simulink model "model_main3"  (R2024b)
settings: Solver=ode4  StartTime=0.0  StopTime=1000  FixedStep=dt  RelTol=1e-3
values from neighbouring files (symbols this model uses):
  dt = 0.01    [model_init.m]
  Iws = diag([1 1 1 1])*0.2274    [model_init.m]
  m_tot = 3300    [model_init.m]
  Omega1_init = 1500*rpm2rad    (= 157.079632679)    [model_init.m]
  Omega2_init = 2500*rpm2rad    (= 261.799387799)    [model_init.m]
  Omega3_init = 1500*rpm2rad    (= 157.079632679)    [model_init.m]
  Omega4_init = 2500*rpm2rad    (= 261.799387799)    [model_init.m]
  qb0 = angle2quat(ag0(1),ag0(2),ag0(3),'ZYX')'    [model_init.m]
  rad2rpm = 1/rpm2rad    (= 9.54929658551)    [model_init.m]
  RCS_F = 1.0    (= 1)    [model_init.m]
  RCS_Pos = [RCS1_POS , RCS2_POS , RCS3_POS , RCS4_POS ,            RCS5_POS , RCS6_POS , RCS7_POS , RCS8_POS ,            RCS9_POS , RCS10_POS, RCS11_POS, RCS12_POS,            RCS13_POS, RCS14_POS, RCS15_POS, RCS16_POS]    [model_init.m]
  RCS_PWM_Freq = 0.1    [model_init.m]
  RCS_Sampling_time = 0.01    [model_init.m]
  RCS_THR_vec = [RCS1_THR , RCS2_THR , RCS3_THR , RCS4_THR,                 RCS5_THR , RCS6_THR , RCS7_THR , RCS8_THR,                 RCS9_THR , RCS10_THR, RCS11_THR, RCS12_THR,                 RCS13_THR, RCS14_THR, RCS15_THR, RCS16_THR]    [model_init.m]
  RW_As = [RW1_Axis,RW2_Axis,RW3_Axis,RW4_Axis]    [model_init.m]
  RW_Omegad_max = RW_t_max    (= 0.5)    [model_init.m]
  SC_Ib = [1843.56  -0.0019  -803.89 ... (first row only)    [model_init.m]
  SC_Kepler = [(6371.2+600)*1000, 0.00221, 0*pi/180, 0*pi/180, 0, deg2rad(270)]    [model_init.m]
  wb0 = deg2rad([-0.3 -0.1 0.2])'    [model_init.m]
undefined symbols (not defined in the file or in its folder): RS_Max_Speed, TC_Kepler
libraries: simulink x16, simulink_extras x9, sharedtransform x6, aerolibutil x4
settings Model: PacingRate=1.100000  Creator=yhj2019  LastModifiedBy=ASCL
settings DebuggingCC: UnderSpecifiedDimensionMsg=warning
settings RTWCC: GPUComputeCapability=3.5

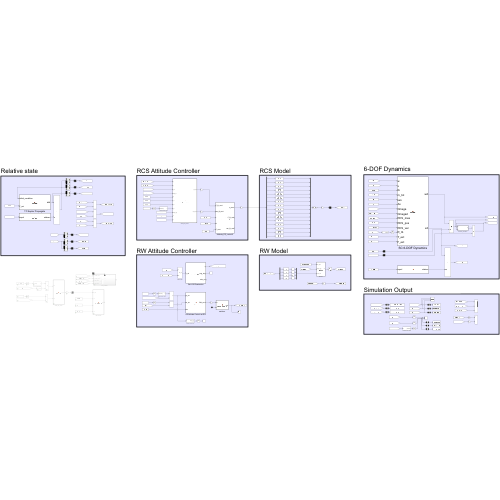
[thumbnail: Simulink's stored preview of the top-level diagram]
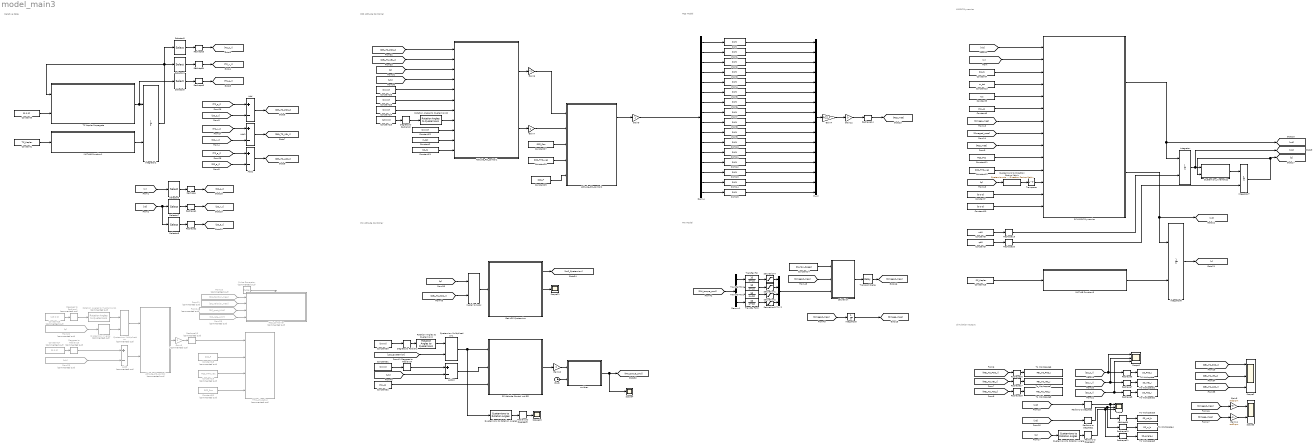
== system model_main3 ==
  note: Relative state
  note: RW Model
  note: RW Attitude Controller
  note: RCS Model
  note: Simulation Output
  note: RCS Attitude Controller
  note: 6-DOF Dynamics
  Add{,1..2,10} (4 alike) : Sum  Inputs=+-
  Add3 : Sum  Commented=on  Inputs=+-
  Attitude_PD_control : MATLAB Function  Commented=on  TreatAsAtomicUnit=on
  Attitude_PD_control1 : MATLAB Function  TreatAsAtomicUnit=on
  Attitude_PD_control2 : MATLAB Function  TreatAsAtomicUnit=on
  Clock : Clock
  Constant1 : Constant  Value=TC_Kepler
  Constant{3,7,10,22,24..25} (6 alike) : Constant  Value=[0 0 0]'
  Constant11 : Constant  Value=RCS_Pos
  Constant12 : Constant  Value=RCS_THR_vec
  Constant13 : Constant  Value=m_tot
  Constant14 : Constant  Value=RS_Max_Speed
  Constant15 : Constant  Value=SC_Kepler
  Constant16 : Constant  Commented=on  Value=[45 0 0]
  Constant17 : Constant  Commented=on  Value=[0 0 0]
  Constant18 : Constant  Commented=on  Value=RCS_F
  Constant19 : Constant  Commented=on  Value=RCS_THR_vec
  Constant2 : Constant  Value=m_tot
  Constant20 : Constant  Commented=on  Value=RCS_Pos
  Constant21 : Constant  Value=SC_Ib
  Constant23 : Constant  Value=[45 0 0]
  Constant26 : Constant  Value=[3 0 0]'
  Constant27 : Constant  Value=RCS_Pos
  Constant28 : Constant  Value=RCS_THR_vec
  Constant29 : Constant  Value=RCS_F
  Constant30 : Constant  Value=[0 0 0]
  Constant31 : Constant  Value=[0 0 0]
  Constant32 : Constant  Value=RW_As
  Constant4 : Constant  Value=SC_Ib
  Constant5 : Constant  Value=Iws
  Constant6 : Constant  Value=RW_As
  Constant8 : Constant  Value=wb0
  Constant9 : Constant  Value=qb0
  Degrees to Radians : simulink_extras/Transformations/Degrees to Radians
  Degrees to Radians1 : simulink_extras/Transformations/Degrees to Radians  Commented=on
  Degrees to Radians2 : simulink_extras/Transformations/Degrees to Radians
  Degrees to Radians3 : simulink_extras/Transformations/Degrees to Radians  Commented=on
  Degrees to Radians4 : simulink_extras/Transformations/Degrees to Radians
  Demux : Demux  Outputs=16
  Demux1 : Demux
  From10 : From  Commented=on  GotoTag=SC_Position_mea  TagVisibility=global
  From11 : From  Commented=on  GotoTag=SC_Velocity_mea  TagVisibility=global
  From22 : From  Commented=on  GotoTag=q
  From23 : From  Commented=on  GotoTag=wb
  From24 : From  Commented=on  GotoTag=SC_quat_LVLH  TagVisibility=global
  From25 : From  Commented=on  GotoTag=SC_rate_LVLH  TagVisibility=global
  Gain10 : Gain
  Gain11 : Gain  Gain=rad2rpm
  Gain12 : Gain  Gain=0
  Gain4 : Gain  Gain=RCS_F
  Gain5 : Gain  Commented=on
  Gain6 : Gain  Gain=-1
  Gain7 : Gain
  Gain8 : Gain  Gain=rad2rpm
  Gain9 : Gain
  Get LOS Quaternion : MATLAB Function  TreatAsAtomicUnit=on
  Inetial to body : aerolibutil/Quaternion Rotation
  Integrator : Integrator  InitialConditionSource=external  InitialCondition=wb0
  Integrator1 : Integrator  InitialConditionSource=external  InitialCondition=[-7000 0 0 0 -9.175045 0 5233.5]'
  Integrator3 : Integrator  InitialCondition=[Omega1_init Omega2_init Omega3_init Omega4_init]'
  Integrator7 : Integrator  InitialConditionSource=external
  Integrator8 : Integrator  InitialConditionSource=external  InitialCondition=[-7000 0 0 0 -9.175045 0 5233.5]'
  MATLAB Function1 : MATLAB Function  TreatAsAtomicUnit=on
  MATLAB Function3 : MATLAB Function  TreatAsAtomicUnit=on
  Mux1 : Mux
  Mux2 : Mux  Inputs=16
  PWM{,1..15} (16 alike) : simulink/Discontinuities/PWM  DisableCoverage=on  Period=RCS_PWM_Freq  InitialDelay=0  DisallowZeroDutyCycle=off  RunAtFixedTimeIntervals=on  SampleTime=RCS_Sampling_time
  Pulse Generator : DiscretePulseGenerator  Commented=on  PulseType=Time based  Period=0.2  PulseWidth=50
  Quaternion Inverse : aerolibutil/Quaternion Inverse  Commented=on
  Quaternion Multiplication : aerolibutil/Quaternion Multiplication  Commented=on
  Quaternion Multiplication1 : aerolibutil/Quaternion Multiplication
  Quaternion_Kinematics : MATLAB Function  TreatAsAtomicUnit=on
  Quaternions to Direction Cosine Matrix : sharedtransform/Quaternions to  Direction Cosine Matrix  aMode=aMode
      settings: LibrarySourceBlock=|
      | aerolibtransform2/Quaternions to
      | Direction Cosine Matrix
  Quaternions to Rotation Angles : sharedtransform/Quaternions to Rotation Angles  rotationOrder=ZYX  aMode=aMode
  Quaternions to Rotation Angles1 : sharedtransform/Quaternions to Rotation Angles  rotationOrder=ZYX  aMode=aMode
  RCS_Controller : Subsystem  Commented=on
  Radians to Degrees{,1..2,5} (4 alike) : simulink_extras/Transformations/Radians to Degrees
  Reshape{,1..5,14,19..20} (9 alike) : Reshape  OutputDimensionality=Column vector (2-D)
  Reshape{6..11,16..18} (9 alike) : Reshape  OutputDimensionality=Row vector (2-D)
  Reshape15 : Reshape  Commented=on  OutputDimensionality=Column vector (2-D)
  Rotation Angles to Quaternions : sharedtransform/Rotation Angles to Quaternions  rotationOrder=ZYX  aMode=aMode
  Rotation Angles to Quaternions1 : sharedtransform/Rotation Angles to Quaternions  Commented=on  rotationOrder=ZYX  aMode=aMode
  Rotation Angles to Quaternions2 : sharedtransform/Rotation Angles to Quaternions  rotationOrder=ZYX  aMode=aMode
  SC 6-DOF Dynamics : MATLAB Function  TreatAsAtomicUnit=on
  SS Attitude Control wrt ECI : MATLAB Function  TreatAsAtomicUnit=on
  Saturation{1..4} (4 alike) : Saturate  UpperLimit=RW_Omegad_max  LowerLimit=-RW_Omegad_max
  Scope : Scope  NumInputPorts=3
  Scope1 : Scope  NumInputPorts=3
  Scope11 : Scope
  Scope13 : Scope
  Scope2 : Scope  NumInputPorts=3
  Scope3 : Scope  NumInputPorts=2
  Scope4 : Scope
  Selector3 : Selector  InputPortWidth=6  IndexOptions=Index vector (dialog)  Indices=[1 2 3]  OutputSizes=1
  Selector4 : Selector  InputPortWidth=6  IndexOptions=Index vector (dialog)  Indices=[4 5 6]  OutputSizes=1
  Selector5 : Selector  InputPortWidth=6  IndexOptions=Index vector (dialog)  Indices=[4 5 6]  OutputSizes=1
  Selector6 : Selector  InputPortWidth=6  IndexOptions=Index vector (dialog)  Indices=[1 2 3]  OutputSizes=1
  Selector7 : Selector  InputPortWidth=6  IndexOptions=Index vector (dialog)  Indices=[1 2 3]  OutputSizes=1
  Selector8 : Selector  InputPortWidth=6  IndexOptions=Index vector (dialog)  Indices=[4 5 6]  OutputSizes=1
  TC Kepler Propagate : MATLAB Function  TreatAsAtomicUnit=on
  THR_Allocation : MATLAB Function  Commented=on  TreatAsAtomicUnit=on
  To Workspace : ToWorkspace  VariableName=SS_POS_I  SampleTime=-1
      settings: Save2DSignal=2-D array (concatenate along first dimension)
  To Workspace1 : ToWorkspace  VariableName=SS_VEL_I  SampleTime=-1
      settings: Save2DSignal=2-D array (concatenate along first dimension)
  To Workspace2 : ToWorkspace  VariableName=SS_ACC_I  SampleTime=-1
      settings: Save2DSignal=2-D array (concatenate along first dimension)
  To Workspace3 : ToWorkspace  VariableName=SS_wd_b  SampleTime=-1
      settings: Save2DSignal=2-D array (concatenate along first dimension)
  To Workspace4 : ToWorkspace  VariableName=SS_w_b  SampleTime=-1
      settings: Save2DSignal=2-D array (concatenate along first dimension)
  To Workspace5 : ToWorkspace  VariableName=SS_angle_I  SampleTime=-1
      settings: Save2DSignal=2-D array (concatenate along first dimension)
  To Workspace6 : ToWorkspace  VariableName=REL_TS_POS_I  SampleTime=-1
      settings: Save2DSignal=2-D array (concatenate along first dimension)
  To Workspace7 : ToWorkspace  VariableName=REL_TS_VEL_I  SampleTime=-1
      settings: Save2DSignal=2-D array (concatenate along first dimension)
  To Workspace8 : ToWorkspace  VariableName=REL_TS_ACC_I  SampleTime=-1
      settings: Save2DSignal=2-D array (concatenate along first dimension)
  Transfer Fcn{,1..3} (4 alike) : TransferFcn  Numerator=[10]  Denominator=[1 10]
  Transport Delay : TransportDelay  DelayTime=dt  InitialOutput=[0 0 0 0]'
  Transpose : Math  Operator=transpose
  saturation : MATLAB Function  TreatAsAtomicUnit=on
  swicher : MATLAB Function  TreatAsAtomicUnit=on
  wires:
  Constant1/1 -> MATLAB Function1/1(kepel)
  TC Kepler Propagate/1(dfdt) -> Selector5/1, Integrator1/1
  MATLAB Function1/1(statvec) -> Integrator1/2
  Integrator1/1 -> Selector3/1, TC Kepler Propagate/1(initial_condition), Selector4/1
  Constant3/1 -> TC Kepler Propagate/2(F_eci)
  Selector5/1 -> Reshape5/1
  Selector4/1 -> Reshape4/1
  Selector3/1 -> Reshape3/1
  Reshape4/1 -> [TS_v_I]
  Reshape5/1 -> [TS_a_I]
  Reshape3/1 -> [TS_p_I]
  Reshape6/1 -> To Workspace/1
  Reshape7/1 -> To Workspace1/1
  Reshape8/1 -> To Workspace2/1
  [TS_p_I] -> Add/1
  [SS_p_I] -> Add/2
  [SS_v_I] -> Add1/2
  [TS_v_I] -> Add1/1
  [SS_a_I] -> Add2/2
  [TS_a_I] -> Add2/1
  Add/1 -> [REL_TS_POS_I]
  Add1/1 -> [REL_TS_VEL_I]
  Add2/1 -> [REL_TS_ACC_I]
  Constant4/1 -> SC 6-DOF Dynamics/3(Ib)
  Constant5/1 -> SC 6-DOF Dynamics/5(Iws)
  SC 6-DOF Dynamics/1(wd) -> Integrator/1, [wd]
  [wb] -> SC 6-DOF Dynamics/1(w)
  Constant6/1 -> SC 6-DOF Dynamics/6(As)
  Constant7/1 -> SC 6-DOF Dynamics/13(T_ext)
  [Omega_mea] -> SC 6-DOF Dynamics/7(Omega)
  [Omegad_mea] -> SC 6-DOF Dynamics/8(Omegad)
  Quaternion_Kinematics/1(qd) -> Integrator7/1
  Constant8/1 -> Reshape19/1
  Constant9/1 -> Reshape20/1
  Quaternions to Rotation Angles/1 -> Radians to Degrees2/1
  [wd] -> Radians to Degrees/1
  [wb] -> Radians to Degrees1/1
  Radians to Degrees/1 -> Reshape9/1, Scope/1
  Radians to Degrees1/1 -> Reshape10/1, Scope/2
  Radians to Degrees2/1 -> Reshape11/1, Scope/3
  [q] -> Quaternions to Rotation Angles/1
  Constant10/1 -> SC 6-DOF Dynamics/14(F_ext)
  Constant13/1 -> SC 6-DOF Dynamics/4(m_tot)
  [q] -> Quaternions to Direction Cosine Matrix/1
  Quaternions to Direction Cosine Matrix/1 -> Transpose/1
  [SS_v_I] -> Scope1/2, Reshape7/1
  Transpose/1 -> SC 6-DOF Dynamics/12(R_Ib)
  Reshape9/1 -> To Workspace3/1
  Reshape10/1 -> To Workspace4/1
  Reshape11/1 -> To Workspace5/1
  Constant15/1 -> MATLAB Function3/1(kepel)
  MATLAB Function3/1(statvec) -> Integrator8/2
  SC 6-DOF Dynamics/2(xd) -> Integrator8/1, [xd]
  Integrator8/1 -> [x]
  Selector8/1 -> Reshape2/1
  Selector6/1 -> Reshape/1
  [xd] -> Selector8/1, Selector7/1
  [x] -> Selector6/1
  Selector7/1 -> Reshape1/1
  [x] -> SC 6-DOF Dynamics/2(x)
  Constant11/1 -> SC 6-DOF Dynamics/10(RCS_pos)
  Constant12/1 -> SC 6-DOF Dynamics/11(RCS_vec)
  Demux/1 -> PWM/1
  Demux/2 -> PWM1/1
  Demux/3 -> PWM2/1
  Demux/4 -> PWM3/1
  Demux/8 -> PWM7/1
  Demux/5 -> PWM4/1
  Demux/6 -> PWM5/1
  Demux/7 -> PWM6/1
  Demux/14 -> PWM13/1
  Demux/13 -> PWM12/1
  Demux/15 -> PWM14/1
  Demux/12 -> PWM11/1
  Demux/16 -> PWM15/1
  Demux/9 -> PWM8/1
  Demux/10 -> PWM9/1
  Demux/11 -> PWM10/1
  Reshape14/1 -> [RCS_mea]
  PWM/1 -> Mux2/1
  Mux2/1 -> Gain4/1
  PWM1/1 -> Mux2/2
  PWM2/1 -> Mux2/3
  PWM3/1 -> Mux2/4
  PWM4/1 -> Mux2/5
  PWM5/1 -> Mux2/6
  PWM6/1 -> Mux2/7
  PWM7/1 -> Mux2/8
  PWM8/1 -> Mux2/9
  PWM9/1 -> Mux2/10
  PWM10/1 -> Mux2/11
  PWM11/1 -> Mux2/12
  PWM12/1 -> Mux2/13
  PWM13/1 -> Mux2/14
  PWM14/1 -> Mux2/15
  PWM15/1 -> Mux2/16
  [RCS_mea] -> SC 6-DOF Dynamics/9(RCS_mea)
  Gain4/1 -> Gain12/1
  From11/1 -> RCS_Controller/2(SC_Velocity_mea)
  From25/1 -> RCS_Controller/4(SC_rate_LVLH)
  From10/1 -> RCS_Controller/1(SC_Position_mea)
  Pulse Generator/1 -> RCS_Controller/Trigger
  From24/1 -> RCS_Controller/3(SC_quat_LVLH)
  From22/1 -> Quaternion Inverse/1
  Degrees to Radians3/1 -> Add3/1
  Constant18/1 -> THR_Allocation/2(F_on)
  Quaternion Inverse/1 -> Quaternion Multiplication/2
  Quaternion Multiplication/1 -> Attitude_PD_control/1(q_err)
  Constant20/1 -> THR_Allocation/4(r_thr)
  Reshape15/1 -> THR_Allocation/1(tau_cmd)
  From23/1 -> Add3/2
  Attitude_PD_control/1(u_torq) -> Gain5/1
  Degrees to Radians1/1 -> Rotation Angles to Quaternions1/1
  Constant17/1 -> Degrees to Radians3/1
  Rotation Angles to Quaternions1/1 -> Quaternion Multiplication/1
  Constant19/1 -> THR_Allocation/3(f)
  Gain5/1 -> Reshape15/1
  Add3/1 -> Attitude_PD_control/2(w_err)
  Constant16/1 -> Degrees to Radians1/1
  Reshape/1 -> [SS_p_I]
  Reshape1/1 -> [SS_v_I]
  Reshape2/1 -> [SS_a_I]
  [REL_TS_POS_I] -> Reshape16/1
  [REL_TS_VEL_I] -> Reshape17/1
  [REL_TS_ACC_I] -> Reshape18/1
  Reshape16/1 -> To Workspace6/1
  Reshape17/1 -> To Workspace7/1
  Reshape18/1 -> To Workspace8/1
  Attitude_PD_control1/1(F_B_cmd) -> Gain6/1
  Attitude_PD_control1/2(tau_B_cmd) -> Gain7/1
  Attitude_PD_control2/1(u_pwm) -> Gain9/1
  Constant21/1 -> Attitude_PD_control1/11(J)
  Constant2/1 -> Attitude_PD_control1/10(m)
  Constant22/1 -> Attitude_PD_control1/9(omega_d_B)
  Constant23/1 -> Degrees to Radians2/1
  Degrees to Radians2/1 -> Rotation Angles to Quaternions2/1
  Rotation Angles to Quaternions2/1 -> Attitude_PD_control1/8(q_d)
  Constant24/1 -> Attitude_PD_control1/7(a_d)
  Constant25/1 -> Attitude_PD_control1/6(v_d)
  Constant26/1 -> Attitude_PD_control1/5(r_d)
  [wb] -> Attitude_PD_control1/4(omega_B)
  [q] -> Attitude_PD_control1/3(q_IB)
  [REL_TS_POS_I] -> Attitude_PD_control1/1(r_I)
  Gain6/1 -> Attitude_PD_control2/1(F_B_cmd)
  Constant27/1 -> Attitude_PD_control2/3(r)
  Constant28/1 -> Attitude_PD_control2/4(d)
  Constant29/1 -> Attitude_PD_control2/5(F_max)
  [REL_TS_POS_I] -> Scope2/1
  [REL_TS_VEL_I] -> Scope2/2
  [REL_TS_ACC_I] -> Scope2/3
  Gain7/1 -> Attitude_PD_control2/2(tau_B_cmd)
  [REL_TS_VEL_I] -> Attitude_PD_control1/2(v_I)
  [wb] -> Add10/2
  Clock/1 -> swicher/2(t)
  Rotation Angles to Quaternions/1 -> Quaternion Multiplication1/1
  Quaternions to Rotation Angles1/1 -> Radians to Degrees5/1
  Get LOS Quaternion/2(ang_deg) -> Scope11/1
  Radians to Degrees5/1 -> Scope13/1
  Degrees to Radians4/1 -> Add10/1
  Constant32/1 -> SS Attitude Control wrt ECI/3(As)
  Degrees to Radians/1 -> Rotation Angles to Quaternions/1
  Quaternion Multiplication1/1 -> SS Attitude Control wrt ECI/1(q_err), Quaternions to Rotation Angles1/1
  Get LOS Quaternion/1(q) -> [LoS_Quaternion]
  Add10/1 -> SS Attitude Control wrt ECI/2(w_err)
  [LoS_Quaternion] -> Quaternion Multiplication1/2
  Constant30/1 -> Degrees to Radians/1
  Constant31/1 -> Degrees to Radians4/1
  [q] -> Inetial to body/1
  Inetial to body/1 -> Get LOS Quaternion/1(r_rel)
  SS Attitude Control wrt ECI/1(RW_cmd) -> Gain10/1
  [REL_TS_POS_I] -> Inetial to body/2
  Gain9/1 -> Demux/1
  Gain10/1 -> swicher/1(in)
  Gain8/1 -> Scope3/1
  Gain11/1 -> Scope3/2
  Reshape19/1 -> Integrator/2
  Reshape20/1 -> Integrator7/2
  Gain12/1 -> Reshape14/1
  Demux1/1 -> Transfer Fcn/1
  Demux1/4 -> Transfer Fcn3/1
  Demux1/2 -> Transfer Fcn1/1
  Demux1/3 -> Transfer Fcn2/1
  Transfer Fcn/1 -> Saturation4/1
  Transfer Fcn1/1 -> Saturation1/1
  Transfer Fcn2/1 -> Saturation2/1
  Transfer Fcn3/1 -> Saturation3/1
  saturation/1(res) -> Transport Delay/1
  [Omegad_mea] -> Integrator3/1
  Integrator3/1 -> [Omega_mea]
  Integrator/1 -> [wb], Quaternion_Kinematics/1(w)
  Integrator7/1 -> [q], Quaternion_Kinematics/2(q)
  swicher/1(out) -> Scope4/1, [RW_torque_cmd]
  [Omegad_mea] -> Gain8/1
  [Omega_mea] -> Gain11/1
  [RW_torque_cmd] -> Demux1/1
  Transport Delay/1 -> [Omegad_mea]
  Saturation3/1 -> Mux1/4
  Saturation1/1 -> Mux1/2
  Saturation4/1 -> Mux1/1
  Saturation2/1 -> Mux1/3
  Mux1/1 -> saturation/3(torque_cmd)
  [Omegad_mea] -> saturation/2(Omega_mea)
  Constant14/1 -> saturation/1(max_speed)
  [SS_p_I] -> Scope1/1, Reshape6/1
  [SS_a_I] -> Scope1/3, Reshape8/1

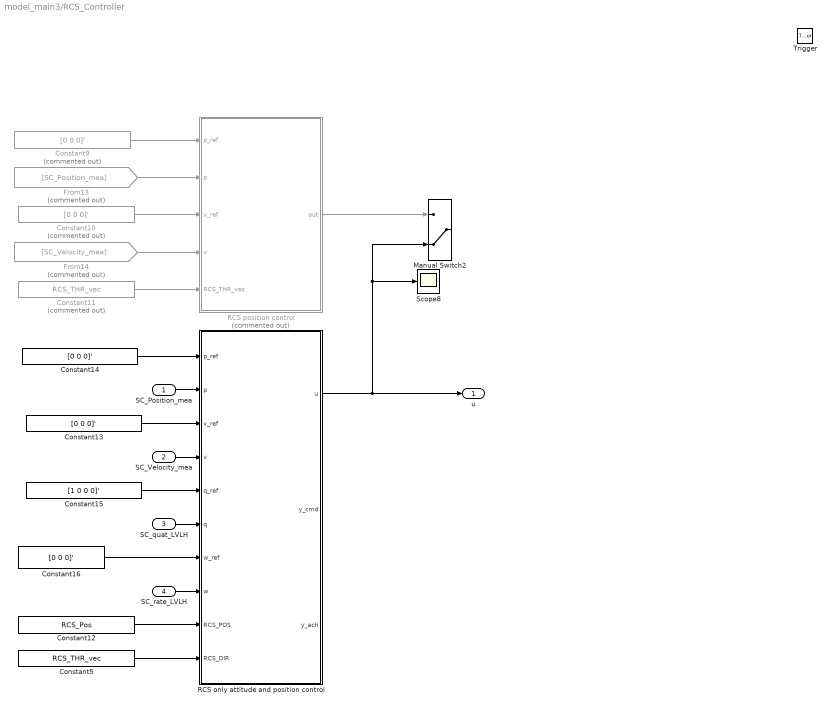
== system model_main3/RCS_Controller ==
  SC_Position_mea : Inport
  SC_Velocity_mea : Inport  Port=2
  SC_quat_LVLH : Inport  Port=3
  SC_rate_LVLH : Inport  Port=4
  Trigger : TriggerPort  TriggerType=either  VariantControl=(inherit)  PortDimensions=1
  Constant10 : Constant  Commented=on  Value=[0 0 0]'
  Constant11 : Constant  Commented=on  Value=RCS_THR_vec
  Constant12 : Constant  Value=RCS_Pos
  Constant13 : Constant  Value=[0 0 0]'
  Constant14 : Constant  Value=[0 0 0]'
  Constant15 : Constant  Value=[1 0 0 0]'
  Constant16 : Constant  Value=[0 0 0]'
  Constant5 : Constant  Value=RCS_THR_vec
  Constant9 : Constant  Commented=on  Value=[0 0 0]'
  From13 : From  Commented=on  GotoTag=SC_Position_mea  TagVisibility=global
  From14 : From  Commented=on  GotoTag=SC_Velocity_mea  TagVisibility=global
  Manual Switch2 : ManualSwitch  CurrentSetting=0
  RCS only attitude and position control : MATLAB Function  TreatAsAtomicUnit=on
  RCS position control : MATLAB Function  Commented=on  TreatAsAtomicUnit=on
  Scope8 : Scope
  u : Outport
  wires:
  Constant5/1 -> RCS only attitude and position control/10(RCS_DIR)
  SC_quat_LVLH/1 -> RCS only attitude and position control/6(q)
  Constant12/1 -> RCS only attitude and position control/9(RCS_POS)
  SC_rate_LVLH/1 -> RCS only attitude and position control/8(w)
  SC_Velocity_mea/1 -> RCS only attitude and position control/4(v)
  From13/1 -> RCS position control/2(p)
  RCS only attitude and position control/1(u) -> Manual Switch2/2, Scope8/1, u/1
  Constant13/1 -> RCS only attitude and position control/3(v_ref)
  Constant15/1 -> RCS only attitude and position control/5(q_ref)
  RCS position control/1(out) -> Manual Switch2/1
  Constant16/1 -> RCS only attitude and position control/7(w_ref)
  Constant10/1 -> RCS position control/3(v_ref)
  Constant9/1 -> RCS position control/1(p_ref)
  Constant11/1 -> RCS position control/5(RCS_THR_vec)
  SC_Position_mea/1 -> RCS only attitude and position control/2(p)
  Constant14/1 -> RCS only attitude and position control/1(p_ref)
  From14/1 -> RCS position control/4(v)

== matlab function model_main3/Attitude_PD_control1 ==
  settings: updateMethod=DISCRETE
  data: F_B_cmd output; r_I input; v_I input; q_IB input; omega_B input; r_d input; v_d input; a_d input; q_d input; omega_d_B input; m input; J input; tau_B_cmd output
function [F_B_cmd, tau_B_cmd] = CTRL_WRENCH_6DOF( ...
    r_I, v_I, q_IB, omega_B, ...
    r_d, v_d, a_d, q_d, omega_d_B, ...
    m, J)
%#codegen
% ============================================================
% Controller block
% Input :
%   r_I      [3x1] current position in inertial frame
%   v_I      [3x1] current velocity in inertial frame
%   q_IB     [4x1] quaternion [qw qx qy qz], Body -> Inertial
%   omega_B  [3x1] current angular velocity in body frame
%
%   r_d      [3x1] desired position in inertial frame
%   v_d      [3x1] desired velocity in inertial frame
%   a_d      [3x1] desired acceleration in inertial frame
%   q_d      [4x1] desired quaternion, Body -> Inertial
%   omega_d_B[3x1] desired angular velocity in body frame
%
%   m        scalar mass
%   J        [3x3] inertia matrix in body frame
%
% Output:
%   F_B_cmd    [3x1] desired total body force
%   tau_B_cmd  [3x1] desired total body torque
% ============================================================

    % -------------------------
    % Quaternion normalize
    % -------------------------
    q_IB = quat_normalize(q_IB);
    q_d  = quat_normalize(q_d);

    % -------------------------
    % Gains (example)
    % -------------------------
    Kp_r = diag([0.010, 0.010, 0.010]);   % position gain
    Kd_r = diag([0.060, 0.060, 0.060]);   % velocity damping

    Kq   = diag([10.0, 10.0, 10.0]);   % attitude gain
    Kw   = diag([6.0,  6.0,  6.0 ]);   % angular-rate damping

    % -------------------------
    % Position control
    % inertial acceleration command
    % -------------------------
    e_r = r_I - r_d;
    e_v = v_I - v_d;

    a_cmd   = a_d - Kp_r * e_r - Kd_r * e_v;
    F_I_cmd = m * a_cmd;

    % Convert inertial force -> body force
    R_IB    = quat_to_rotm(q_IB);
    F_B_cmd = R_IB.' * F_I_cmd;

    % -------------------------
    % Attitude control
    % q_e = q_d^{-1} ⊗ q_IB
    % -------------------------
    q_e = quat_mul(quat_conj(q_d), q_IB);

    % shortest-path quaternion
    if q_e(1) < 0
        q_e = -q_e;
    end

    e_w = omega_B - omega_d_B;

    % PD + gyro compensation
    tau_B_cmd = -Kq * q_e(2:4) ...
                -Kw * e_w ...
                +cross(omega_B, J * omega_B);
end


% ============================================================
% Local helper functions
% ============================================================

function qn = quat_normalize(q)
    n = norm(q);
    if n < 1e-12
        qn = [1;0;0;0];
    else
        qn = q / n;
    end
end

function qc = quat_conj(q)
    qc = [q(1); -q(2); -q(3); -q(4)];
end

function q = quat_mul(q1, q2)
    % Hamilton product
    w1 = q1(1); x1 = q1(2); y1 = q1(3); z1 = q1(4);
    w2 = q2(1); x2 = q2(2); y2 = q2(3); z2 = q2(4);

    q = [ w1*w2 - x1*x2 - y1*y2 - z1*z2;
          w1*x2 + x1*w2 + y1*z2 - z1*y2;
          w1*y2 - x1*z2 + y1*w2 + z1*x2;
          w1*z2 + x1*y2 - y1*x2 + z1*w2 ];
end

function R = quat_to_rotm(q)
    % q = [qw qx qy qz], Body -> Inertial
    qw = q(1); qx = q(2); qy = q(3); qz = q(4);

    R = [1-2*(qy^2+qz^2),   2*(qx*qy-qz*qw),   2*(qx*qz+qy*qw);
         2*(qx*qy+qz*qw),   1-2*(qx^2+qz^2),   2*(qy*qz-qx*qw);
         2*(qx*qz-qy*qw),   2*(qy*qz+qx*qw),   1-2*(qx^2+qy^2)];
end

== matlab function model_main3/Attitude_PD_control2 ==
  settings: updateMethod=DISCRETE
  data: u_pwm output; F_B_cmd input; tau_B_cmd input; F_B_real output; tau_B_real output; r input; d input; F_max input
function [u_pwm, F_B_real, tau_B_real] = ALLOC_THRUSTER_PWM_12(F_B_cmd, tau_B_cmd, r, d, F_max)
%#codegen
% ============================================================
% Allocation block
% Input :
%   F_B_cmd    [3x1] desired total body force
%   tau_B_cmd  [3x1] desired total body torque
%
% Output:
%   u_pwm      [12x1] thruster duty command, 0 ~ 1
%   F_B_real   [3x1] realized body force after allocation
%   tau_B_real [3x1] realized body torque after allocation
%
% Example:
%   12-thruster layout for 6DoF control
%   Replace thruster geometry / Tmax below with your real spacecraft values.
% ============================================================

    % Build 6x12 thruster mapping matrix A
    A = build_thruster_matrix( 16, r, d, F_max);

    % Desired wrench
    w_cmd = [F_B_cmd; tau_B_cmd];

    % Bounded least-squares allocation: 0 <= u <= 1
    u_pwm = bounded_allocator_0_1(A, w_cmd);

    % Realized wrench
    w_real     = A * u_pwm;
    F_B_real   = w_real(1:3);
    tau_B_real = w_real(4:6);
end


% ============================================================
% Thruster layout
% ============================================================
function A = build_thruster_matrix(N, r, d, F_max)
    % --------------------------------------------------------
    % Example spacecraft half-size [m]
    % Replace with your real geometry
    % --------------------------------------------------------
    % L = 0.50;   % lever arm

    % --------------------------------------------------------
    % Max thrust of each thruster [N]
    % Replace with your real thruster max force
    % --------------------------------------------------------
    Tmax = F_max * ones(N,1);

    % --------------------------------------------------------
    % Thruster positions r_i in body frame [m]
    % Each column is one thruster position
    % --------------------------------------------------------
    % r = [ ...
    %      0,   0,   0,   0,   L,  -L,   L,  -L,   L,  -L,   L,  -L;
    %      L,  -L,   L,  -L,   0,   0,   0,   0,   L,   L,  -L,  -L;
    %      L,  -L,  -L,   L,   L,  -L,  -L,   L,   0,   0,   0,   0 ];

    % --------------------------------------------------------
    % Thruster unit directions d_i in body frame
    %
    % T1,T2 : +X
    % T3,T4 : -X
    % T5,T6 : +Y
    % T7,T8 : -Y
    % T9,T10: +Z
    % T11,T12:-Z
    % --------------------------------------------------------
    % d = [ ...
    %      1,   1,  -1,  -1,   0,   0,   0,   0,   0,   0,   0,   0;
    %      0,   0,   0,   0,   1,   1,  -1,  -1,   0,   0,   0,   0;
    %      0,   0,   0,   0,   0,   0,   0,   0,   1,   1,  -1,  -1 ];

    % --------------------------------------------------------
    % Build A = [F; tau], size 6x12
    % --------------------------------------------------------
    A = zeros(6,N);

    for i = 1:N
        f_i       = Tmax(i) * d(:,i);
        tau_i     = cross(r(:,i), f_i);
        A(:,i)    = [f_i; tau_i];
    end
end


% ============================================================
% Bounded allocator: 0 <= u <= 1
% Codegen-friendly fixed-size active-set style
% ============================================================
function u = bounded_allocator_0_1(A, w_cmd)
    N = 16;
    u = zeros(N,1);

    % free_mask(i)=true means this thruster is still free to solve
    free_mask = true(N,1);

    lambda = 1e-8;   % small damping

    for iter = 1:(N+1)

        % Residual after fixed/saturated thrusters
        w_res = w_cmd;
        for i = 1:N
            if ~free_mask(i)
                w_res = w_res - A(:,i) * u(i);
            end
        end

        % Collect free columns into Af (fixed-size construction)
        Af  = zeros(6,N);
        idx = zeros(N,1);
        nf  = 0;

        for i = 1:N
            if free_mask(i)
                nf = nf + 1;
                idx(nf) = i;
                Af(:,nf) = A(:,i);
            end
        end

        if nf == 0
            break;
        end

        % Minimum-norm damped solution on free set
        M       = Af * Af.' + lambda * eye(6);
        uf_full = Af.' * (M \ w_res);   % size Nx1, only first nf entries used

        % Put candidate solution into u
        for k = 1:nf
            i = idx(k);
            u(i) = uf_full(k);
        end

        % Check bounds and fix saturated variables
        violated = false;
        for k = 1:nf
            i = idx(k);

            if u(i) < 0
                u(i) = 0;
                free_mask(i) = false;
                violated = true;

            elseif u(i) > 1
                u(i) = 1;
                free_mask(i) = false;
                violated = true;
            end
        end

        if ~violated
            break;
        end
    end

    % Final clipping
    for i = 1:N
        if u(i) < 0
            u(i) = 0;
        elseif u(i) > 1
            u(i) = 1;
        end
    end
end

== matlab function model_main3/saturation ==
  data: max_speed input; res output; Omega_mea input; torque_cmd input
function res  = saturation(max_speed, Omega_mea, torque_cmd)

Omega1_mea = Omega_mea(1);
Omega2_mea = Omega_mea(2);
Omega3_mea = Omega_mea(3);
Omega4_mea = Omega_mea(4);

if abs(Omega1_mea)> max_speed
    res1 = 0;
else
    res1 = torque_cmd(1);
end

if abs(Omega2_mea)>max_speed
    res2 = 0;
else
    res2 = torque_cmd(2);
end

if abs(Omega3_mea)>max_speed
    res3 = 0;
else
    res3 = torque_cmd(3);
end

if abs(Omega4_mea)>max_speed
    res4 = 0;
else
    res4 = torque_cmd(4);
end

res = [res1,res2,res3,res4]';

end

== matlab function model_main3/Get LOS Quaternion ==
  data: r_rel input; q output; ang_deg output; axis_rot output
function [q, ang_deg, axis_rot] = boresight_to_target_quat(r_rel)
%#codegen
% ============================================================
% boresight_to_target_quat
%
% Input:
%   r_rel    [3x1] : relative position vector
%
% Output:
%   q        [4x1] : quaternion [w; x; y; z]
%                    rotating boresight [1;0;0] to r_rel direction
%   ang_deg  [1x1] : rotation angle in degrees
%   axis_rot [3x1] : rotation axis (unit vector)
%
% Notes:
%   - boresight reference is fixed as [1; 0; 0]
%   - quaternion is scalar-first
%   - handles parallel / anti-parallel edge cases
% ============================================================

    % Reference boresight
    b_ref = [1; 0; 0];

    % Small threshold
    eps_val = 1e-12;

    % Check input norm
    r_norm = norm(r_rel);
    if r_norm < eps_val
        % Undefined direction
        q = [1; 0; 0; 0];
        ang_deg = 0;
        axis_rot = [1; 0; 0];
        return;
    end

    % Normalize target direction
    v = r_rel / r_norm;
    u = b_ref;

    % Dot product
    c = dot(u, v);
    c = max(min(c, 1.0), -1.0);   % numerical safety

    % Case 1: same direction
    if c > 1 - 1e-10
        q = [1; 0; 0; 0];
        ang_deg = 0;
        axis_rot = [1; 0; 0];
        return;
    end

    % Case 2: opposite direction
    if c < -1 + 1e-10
        % Need 180 deg rotation about any axis orthogonal to [1;0;0]
        % Choose y-axis
        axis_rot = [0; 1; 0];
        q = [0; axis_rot];   % cos(pi/2)=0, sin(pi/2)=1
        ang_deg = 180;
        return;
    end

    % General case
    cross_uv = cross(u, v);

    % Robust quaternion from two vectors:
    % q = [1 + dot(u,v); cross(u,v)] then normalize
    q = [1 + c;
         cross_uv(1);
         cross_uv(2);
         cross_uv(3)];

    q = q / norm(q);

    % Rotation angle
    ang_rad = 2 * acos(q(1));
    ang_deg = ang_rad * 180 / pi;

    % Rotation axis
    s = sqrt(1 - q(1)^2);
    if s < 1e-10
        axis_rot = [1; 0; 0];
    else
        axis_rot = q(2:4) / s;
    end
end

== matlab function model_main3/Attitude_PD_control ==
  settings: updateMethod=DISCRETE
  data: u_torq output; q_err input; w_err input
function u_torq = att_pd_control(q_err, w_err)

persistent first_flg
persistent I_save

dt = 0.01;

if isempty(first_flg)
    first_flg = 1;
    I_save = [0 0 0]';
end

K1 = 10.1*diag([1 1 1]);
K2 = 8.2*diag([1 1 1]);
K3 = 0.1*diag([1 1 1]);

q_err_ = [q_err(2), q_err(3), q_err(4)]';

u_torq = K1*q_err_ + K2*w_err + K3*I_save;

I_save = I_save + q_err_ * dt;

end

== matlab function model_main3/THR_Allocation ==
  data: pwm output; tau_cmd input; F_on input; f input; r_thr input
function pwm = RCS_Torque2PWM(tau_cmd, F_on, f, r_thr)
%#codegen
% ============================================================
% Minimal RCS allocation: torque command -> PWM duty (0..1)
%   tau ≈ sum_i r_i x (f_i * F_on_i * pwm_i)
%
% Inputs:
%   tau_cmd [3x1]
%   F_on    scalar or [12x1]
%   f       [3x12]  (columns are unit vectors)
%   r_thr   [3x12]  (columns are position vectors wrt CoM)
%
% Output:
%   pwm     [12x1] duty in [0,1]
% ============================================================
N = 16;
% F_on -> 12x1
if isscalar(F_on)
    Fon = F_on * ones(N,1);
else
    Fon = F_on(:);
end

% Build effectiveness matrix B (3x12): tau = B * pwm
B = zeros(3,N);
for i = 1:N
    Fi = Fon(i);
    B(:,i) = cross3(r_thr(:,i), f(:,i) * Fi);  % torque from pwm=1
end

% Unconstrained least-squares solution (minimum-norm)
pwm = B' * ((B*B') \ tau_cmd);

% Clamp to [0,1]
for i=1:N
    if pwm(i) < 0, pwm(i) = 0; end
    if pwm(i) > 1, pwm(i) = 1; end
end

end

function c = cross3(a,b)
c = [ a(2)*b(3) - a(3)*b(2);
      a(3)*b(1) - a(1)*b(3);
      a(1)*b(2) - a(2)*b(1) ];
end

== matlab function model_main3/Quaternion_Kinematics ==
  data: w input; qd output; q input
function qd = fcn(w,q)

F_q = (1/2)*[0 -w(1) -w(2) -w(3);
       w(1) 0 w(3) -w(2);
       w(2) -w(3) 0 w(1);
       w(3) w(2) -w(1) 0];

qd = F_q*q;

end

== matlab function model_main3/SS Attitude Control wrt ECI ==
  settings: updateMethod=DISCRETE
  data: q_err input; RW_cmd output; w_err input; As input
function RW_cmd  = Att_PD_Control(q_err, w_err, As)

persistent I_save
persistent flg

if isempty(flg)
    flg = 1;
    I_save = [0 0 0]';
end

K1 = 100.0*diag([1 1 1]);
K2 = 2000.0*diag([1 1 1]);
K3 = 1.0*diag([1 1 1]);

q_e_v = [q_err(2), q_err(3), q_err(4)]';

u = K1*q_e_v + K2*w_err + K3*I_save;

RW_cmd = pinv(As)*-u;

I_save = I_save + (q_e_v*0.01);

end

== matlab function model_main3/swicher ==
  settings: updateMethod=DISCRETE
  data: out output; in input; t input
function out  =  rcs_attitude_allocator_only(in, t)


if t>2
    out = in;
else
    out = 0*in;

end

end

== matlab function model_main3/MATLAB Function1 ==
  data: kepel input; statvec output
function statvec  = kepel_statvec (kepel)
%  [statvec] = kepel_statvec (kepel)
%	The function kepel_statvec transforms the keplerian
%	elements kepel into the corresponding state vector in
%	the same reference system.
%
% Input:
%	kepel
% 		vector containing the keplerian elements:
%		(1) - semimajor axis of the orbit in meters.
%		(2) - eccentricity.
%		(3) - inclinatsion in radians.
%		(4) - right ascension of ascending node in radians.
%		(5) - argument of perigee in radians.
%		(6) - mean anomaly in radians.
% Output:
%	statvec
%  		state vector in meters and meters/second.
%
% Authors:
%	Helio K. Kuga;
%	Valder M. Medeiros;
%	Valdemir Carrara		february/80		version 1.0
%	Valdemir Carrara		july 2005		(C version)
%   Valdemir Carrara            March/09        Matlab

EARTH_GRAVITY	= 3.9860064e+14;		% Earth's gravitational constant (m**3/s**2)

a    = kepel(1);	% semi-major axis
exc  = kepel(2);	% eccentricity

c1   = sqrt(1. - exc*exc);

%     rotation matrix

orb2iner = rotmaz(-kepel(4))*rotmax(-kepel(3))*rotmaz(-kepel(5));

%     Kepler's equation

E    = kepler(kepel(6), exc);

sE   = sin(E);
cE   = cos(E);
c3   = sqrt(EARTH_GRAVITY/a)/(1. - exc*cE);

%     state vector

statvec = [[a*(cE - exc), a*c1*sE, 0]*orb2iner', [-c3*sE, c1*c3*cE, 0]*orb2iner'];

end

function [rot_mat] = rotmax (angle)
% [rot_mat] = rotmax (angle)
%   To obtain the rotation matrix around the X axis given the
%   rotation angle.
% inputs:
%   angle
%       rotation angle, in radians.
% outputs:
%   rot_mat
%       rotation matrix (3, 3)
%

% Valdemir Carrara, Sep, 1998

coan    =  cos(angle);
sian    =  sin(angle);

rot_mat =  [1, 0, 0; 0, coan, sian; 0, -sian, coan];

end

function [rot_mat] = rotmay (angle)
% [rot_mat] = rotmay (angle)
%   To obtain the rotation matrix around the Y axis given the
%   rotation angle.
% inputs:
%   angle
%       rotation angle, in radians.
% outputs:
%   rot_mat
%       rotation matrix (3, 3)
%

% Valdemir Carrara, Sep, 1998


coan    =  cos(angle);
sian    =  sin(angle);

rot_mat =  [coan, 0, -sian; 0, 1, 0; sian, 0, coan];

end

function [rot_mat] = rotmaz (angle)
% [rot_mat] = rotmaz (angle)
%   To obtain the rotation matrix around the Z axis given the
%   rotation angle.
% inputs:
%   angle
%       rotation angle, in radians.
% outputs:
%   rot_mat
%       rotation matrix (3, 3)
%

% Valdemir Carrara, Sep, 1998

coan    =  cos(angle);
sian    =  sin(angle);

rot_mat =  [coan, sian, 0; -sian, coan, 0; 0, 0, 1];
end

function [eccentric] = kepler (mean_anomaly, eccentricity)
% [eccentric] = kepler (mean_anomaly, eccentricity)
%	The subroutine kepler finds a solution to the
%	kepler's equation.
%
% Input:
%	mean_anomaly
%		mean anomaly in radians.
%	eccentricity
%		eccentricity.
%
% Output:
%	eccentric
%		eccentric anomaly in radians.
%
% Authors:
%	Valder M. de Medeiros		june/81		version 2.0
%	Valdemir Carrara			july 2005	(C version)
%   Valdemir Carrara            March/09        Matlab

exc2    = eccentricity*eccentricity;
am1     = mod (mean_anomaly, 2*pi);
am2     = am1 + am1;
am3     = am1 + am2;
shoot   = am1 + eccentricity*(1. - 0.125*exc2)*sin(am1) + ...
		0.5*exc2*(sin(am2) + 0.75*eccentricity*sin(am3));
shoot   = mod (shoot, 2*pi);

e1      = 1.0;
ic      = 0;

while ((abs(e1) > 1.e-12) && (ic <= 10)) 
	e1    = (shoot - am1 - eccentricity*sin(shoot)) / ...
			(1.0 - eccentricity*cos(shoot));
    shoot = shoot - e1;
    ic    = ic + 1;
end

if (ic >= 10)
    disp ('warning ** subroutine kepler did not converge in 10 iterations');
end

eccentric = shoot;


end

== matlab function model_main3/TC Kepler Propagate ==
  data: initial_condition input; dfdt output; F_eci input
function dfdt  = eq_propagate(initial_condition, F_eci)
% Lectures_TwoBodyProblem.pdf
% 우주시스템입문 - 도미타 노부유키 eq(7.8) p136
% https://en.wikipedia.org/wiki/Standard_gravitational_parameter
u  = 3.9860064e+14; % earth gravitional parameter
Re = 6378137;      % earth radius [m]

dfdt = zeros(size(initial_condition));

% x=x
% x1=dx/dt
% dx1/dt = d^2(x)/dt

x1 = initial_condition(4); % x1 = dx/dt
y1 = initial_condition(5); % y1 = dy/dt
z1 = initial_condition(6); % z1 = dz/dt
x  = initial_condition(1); % x
y  = initial_condition(2); % y
z  = initial_condition(3); % z

r=sqrt(x^2+y^2+z^2);

% % %   Keplar Motion Equatnion
% % %  => r_dd + u/(r^3)r_ = 0 => r_dd = -u/(r^3)r_
dfdt(1) = x1;
dfdt(2) = y1;
dfdt(3) = z1;
dfdt(4) = -u*x/(r^3) + F_eci(1);
dfdt(5) = -u*y/(r^3) + F_eci(2);
dfdt(6) = -u*z/(r^3) + F_eci(3);

end

== matlab function model_main3/SC 6-DOF Dynamics ==
  data: w input; x input; Ib input; m_tot input; Iws input; As input; Omega input; Omegad input; RCS_mea input; RCS_pos input; RCS_vec input; wd output; R_Ib input; T_ext input; F_ext input; xd output
function [wd, xd]  = eq_propagate(w, x, Ib, m_tot, ...
                                   Iws, As, Omega, Omegad, ...
                                   RCS_mea, RCS_pos, RCS_vec, R_Ib, ...
                                   T_ext, F_ext)
% % 
% 출력 1: 위성 동체 좌표계 각가속도
% 출력 2: 관성좌표계 선가속도

% % 
RW_h = As*Iws*Omega;
RW_hd = As*Iws*Omegad;

% % 
N = 16;
RCS_f = zeros(3,N);
RCS_t = zeros(3,N);

for i = 1:N
    r_i = RCS_pos(:,i);   % position of thruster i
    d_i = RCS_vec(:,i);   % thrust direction of thruster i

    % force contribution
    RCS_f(:,i) = d_i;

    % torque contribution
    RCS_t(:,i) = cross(r_i, d_i);
end
RCS_f_total = RCS_f * RCS_mea;  % [3x1]
RCS_t_total = RCS_t * RCS_mea;  % [3x1]


%% Rotational Motion
wd = [0 0 0]';
wd = inv(Ib)*(T_ext + RCS_t_total - RW_hd - cross(w, Ib*w + RW_h));

%% Translational Motion

F_I = R_Ib * RCS_f_total;

u  = 3.9860064e+14; % earth gravitional parameter
Re = 6378137;      % earth radius [m]

xd = zeros(size(x));

v1_i = x(4); % x1 = dx/dt
v2_i = x(5); % y1 = dy/dt
v3_i = x(6); % z1 = dz/dt
p1_i = x(1); % x
p2_i = x(2); % y
p3_i = x(3); % z

r=sqrt(p1_i^2+p2_i^2+p3_i^2);

% % %   Keplar Motion Equatnion
% % %  => r_dd + u/(r^3)r_ = 0 => r_dd = -u/(r^3)r_
xd(1) = v1_i;
xd(2) = v2_i;
xd(3) = v3_i;
xd(4) = -u*p1_i/(r^3) + F_I(1) + F_ext(1);
xd(5) = -u*p2_i/(r^3) + F_I(2) + F_ext(2);
xd(6) = -u*p3_i/(r^3) + F_I(3) + F_ext(3);

end

== matlab function model_main3/MATLAB Function3 ==
  data: kepel input; statvec output
function statvec  = kepel_statvec (kepel)
%  [statvec] = kepel_statvec (kepel)
%	The function kepel_statvec transforms the keplerian
%	elements kepel into the corresponding state vector in
%	the same reference system.
%
% Input:
%	kepel
% 		vector containing the keplerian elements:
%		(1) - semimajor axis of the orbit in meters.
%		(2) - eccentricity.
%		(3) - inclinatsion in radians.
%		(4) - right ascension of ascending node in radians.
%		(5) - argument of perigee in radians.
%		(6) - mean anomaly in radians.
% Output:
%	statvec
%  		state vector in meters and meters/second.
%
% Authors:
%	Helio K. Kuga;
%	Valder M. Medeiros;
%	Valdemir Carrara		february/80		version 1.0
%	Valdemir Carrara		july 2005		(C version)
%   Valdemir Carrara            March/09        Matlab

EARTH_GRAVITY	= 3.9860064e+14;		% Earth's gravitational constant (m**3/s**2)

a    = kepel(1);	% semi-major axis
exc  = kepel(2);	% eccentricity

c1   = sqrt(1. - exc*exc);

%     rotation matrix

orb2iner = rotmaz(-kepel(4))*rotmax(-kepel(3))*rotmaz(-kepel(5));

%     Kepler's equation

E    = kepler(kepel(6), exc);

sE   = sin(E);
cE   = cos(E);
c3   = sqrt(EARTH_GRAVITY/a)/(1. - exc*cE);

%     state vector

statvec = [[a*(cE - exc), a*c1*sE, 0]*orb2iner', [-c3*sE, c1*c3*cE, 0]*orb2iner'];

end

function [rot_mat] = rotmax (angle)
% [rot_mat] = rotmax (angle)
%   To obtain the rotation matrix around the X axis given the
%   rotation angle.
% inputs:
%   angle
%       rotation angle, in radians.
% outputs:
%   rot_mat
%       rotation matrix (3, 3)
%

% Valdemir Carrara, Sep, 1998

coan    =  cos(angle);
sian    =  sin(angle);

rot_mat =  [1, 0, 0; 0, coan, sian; 0, -sian, coan];

end

function [rot_mat] = rotmay (angle)
% [rot_mat] = rotmay (angle)
%   To obtain the rotation matrix around the Y axis given the
%   rotation angle.
% inputs:
%   angle
%       rotation angle, in radians.
% outputs:
%   rot_mat
%       rotation matrix (3, 3)
%

% Valdemir Carrara, Sep, 1998


coan    =  cos(angle);
sian    =  sin(angle);

rot_mat =  [coan, 0, -sian; 0, 1, 0; sian, 0, coan];

end

function [rot_mat] = rotmaz (angle)
% [rot_mat] = rotmaz (angle)
%   To obtain the rotation matrix around the Z axis given the
%   rotation angle.
% inputs:
%   angle
%       rotation angle, in radians.
% outputs:
%   rot_mat
%       rotation matrix (3, 3)
%

% Valdemir Carrara, Sep, 1998

coan    =  cos(angle);
sian    =  sin(angle);

rot_mat =  [coan, sian, 0; -sian, coan, 0; 0, 0, 1];
end

function [eccentric] = kepler (mean_anomaly, eccentricity)
% [eccentric] = kepler (mean_anomaly, eccentricity)
%	The subroutine kepler finds a solution to the
%	kepler's equation.
%
% Input:
%	mean_anomaly
%		mean anomaly in radians.
%	eccentricity
%		eccentricity.
%
% Output:
%	eccentric
%		eccentric anomaly in radians.
%
% Authors:
%	Valder M. de Medeiros		june/81		version 2.0
%	Valdemir Carrara			july 2005	(C version)
%   Valdemir Carrara            March/09        Matlab

exc2    = eccentricity*eccentricity;
am1     = mod (mean_anomaly, 2*pi);
am2     = am1 + am1;
am3     = am1 + am2;
shoot   = am1 + eccentricity*(1. - 0.125*exc2)*sin(am1) + ...
		0.5*exc2*(sin(am2) + 0.75*eccentricity*sin(am3));
shoot   = mod (shoot, 2*pi);

e1      = 1.0;
ic      = 0;

while ((abs(e1) > 1.e-12) && (ic <= 10)) 
	e1    = (shoot - am1 - eccentricity*sin(shoot)) / ...
			(1.0 - eccentricity*cos(shoot));
    shoot = shoot - e1;
    ic    = ic + 1;
end

if (ic >= 10)
    disp ('warning ** subroutine kepler did not converge in 10 iterations');
end

eccentric = shoot;


end

== matlab function model_main3/RCS_Controller/RCS only attitude and position control ==
  data: p_ref input; u output; p input; v_ref input; v input; q_ref input; q input; w_ref input; w input; RCS_POS input; RCS_DIR input; y_cmd output; y_ach output
function [u, y_cmd, y_ach] = fcn( ...
                                  p_ref, p, v_ref, v, ...          % position control
                                  q_ref, q, w_ref, w, ...          % attitude control (quat + body rates)
                                  RCS_POS, RCS_DIR)                % thruster geometry
%#codegen
% p, v : 3x1 [m], [m/s]
% q_ref, q : 4x1 quaternion (scalar-first: [qw qx qy qz]')
% w_ref, w : 3x1 [rad/s] (body frame)
% RCS_POS : 3xN position vectors of thrusters wrt CoM [m]
% RCS_DIR : 3xN thrust direction unit vectors [N/A] in body frame
% u : Nx1 thrust commands [N]

% ====== Parameters ======
Tmax = 22;       % [N]
m    = 2000;     % [kg]

% Translational PD gains
Kp_p = 2 * diag([1 1 1]);
Kd_p = 4 * diag([1 1 1]);

% Attitude PD gains (원하시면 사용하신 K1,K2 그대로 넣으셔도 됩니다)
Kq = 0.5 * diag([1 1 1]);    % quaternion-vector part gain
Kw = 2  * diag([1 1 1]);    % angular-rate gain

% (선택) 힘/토크 가중치: 단위/스케일 차이 때문에 보통 넣는 걸 권장합니다.
wF   = 1.0;    % force weight
wTau = 1.0;    % torque weight (필요 시 크게/작게 조정)

% ====== 1) Translation: PD -> F_cmd ======
e_p = p_ref - p;
e_v = v_ref - v;

a_cmd = Kp_p*e_p + Kd_p*e_v;
F_cmd = m * a_cmd;              % 3x1

% ====== 2) Attitude: quaternion error + rate error -> Tau_cmd ======
qe = quat_err_scalar_first(q_ref, q);     % q_err = q_ref ⊗ conj(q)
% 쿼터니언 언와인딩 방지(연속성)
if qe(1) < 0
    qe = -qe;
end
qe_v = qe(2:4);

we = w - w_ref;                 % body rate error (원하시면 w_ref-w 로 바꾸셔도 됨)

% 기본적인 PD 토크(부호는 시스템 정의에 맞게 조정 가능)
Tau_cmd = -(Kq*qe_v + Kw*we);    % 3x1

% ====== 3) Build 6xN allocation matrix B ======
N = size(RCS_DIR, 2);

B = zeros(6, N);
for i = 1:N
    ti = RCS_DIR(:, i);          % 3x1
    ri = RCS_POS(:, i);          % 3x1
    B(1:3, i) = ti;
    B(4:6, i) = cross(ri, ti);
end

% ====== 4) Stack command y = [F; Tau] and solve allocation ======
y_cmd = [wF*F_cmd; wTau*Tau_cmd];      % 6x1
Bw    = [wF*B(1:3,:); wTau*B(4:6,:)];  % weighted B

% 간단 대안: pinv + clip + active-set 반복(툴박스 없이 가능)
u = rcs_allocate_pinv_clip_iter(Bw, y_cmd, Tmax);

y_ach = B*u;    % achieved (unweighted, physical)

end

% ===== Helper: iterative clipped pseudo-inverse allocation =====
function u = rcs_allocate_pinv_clip_iter(B, y, Tmax)
%#codegen
N = size(B,2);

% 초기 해
u = pinv(B) * y;

% active-set 반복: 0 또는 Tmax에 걸린 추력기는 고정하고 나머지만 재해결
MAX_IT = 10;
for k = 1:MAX_IT
    u_prev = u;

    % bounds 적용
    u = max(u, 0);
    u = min(u, Tmax);

    % 자유 변수 마스크
    free = (u > 1e-9) & (u < Tmax - 1e-9);

    if ~any(free)
        break;
    end

    % 고정된 변수 기여를 빼고, 자유 변수만 재계산
    y_res = y - B(:, ~free) * u(~free);
    Bf    = B(:, free);

    uf = pinv(Bf) * y_res;

    u(free) = uf;

    % 수렴 체크
    if norm(u - u_prev) < 1e-6
        break;
    end
end
end

% ===== Helper: quaternion error (scalar-first) =====
function qe = quat_err_scalar_first(q_ref, q)
%#codegen
% qe = q_ref ⊗ conj(q)
qc = [q(1); -q(2); -q(3); -q(4)];

qe = quat_mul_scalar_first(q_ref, qc);
end

function q = quat_mul_scalar_first(q1, q2)
%#codegen
w1=q1(1); x1=q1(2); y1=q1(3); z1=q1(4);
w2=q2(1); x2=q2(2); y2=q2(3); z2=q2(4);

q = [ ...
    w1*w2 - x1*x2 - y1*y2 - z1*z2; ...
    w1*x2 + x1*w2 + y1*z2 - z1*y2; ...
    w1*y2 - x1*z2 + y1*w2 + z1*x2; ...
    w1*z2 + x1*y2 - y1*x2 + z1*w2  ...
    ];
end

== matlab function model_main3/RCS_Controller/RCS position control ==
  data: p_ref input; out output; p input; v_ref input; v input; RCS_THR_vec input
function out = fcn(p_ref, p, v_ref, v, RCS_THR_vec)
% ====== 파라미터 ======
Tmax   = 22;       % [N]
m = 2000;
% pwmMax = 65535;    % 예: 16-bit
% pwmMin = 0;        % 필요하면 최소 구동값 넣기
Kp = 20*diag([1 1 1]);
Kd = 40*diag([1 1 1]);
% ====== 1) PD -> F_cmd ======
e_p = p_ref - p;
e_v = v_ref - v;

a_cmd = Kp*e_p + Kd*e_v;
F_cmd = m * a_cmd;

% ====== 2) Allocation ======
% [u, F_ach] = rcs_allocate_lsqlin(F_cmd, RCS_THR_vec, Tmax); % toolbox 권장
[u, F_ach] = rcs_allocate_pinv_clip(F_cmd, RCS_THR_vec, Tmax); % 간단 대안

% ====== 3) PWM ======
% pwm = thrust_to_pwm(u, Tmax, pwmMax, pwmMin);
out = u./1;
% (디버그)
% disp("F_cmd  = " + mat2str(F_cmd',4))
% disp("F_ach  = " + mat2str(F_ach',4))
% disp("u(N)   = " + mat2str(u',4))
% disp("pwm    = " + mat2str(pwm',4))

end

function [u, F_ach] = rcs_allocate_pinv_clip(F_cmd, RCS_THR_vec, Tmax)
    B = RCS_THR_vec;     % 3xN
    u = pinv(B) * F_cmd; % unconstrained

    % Thruster는 보통 단방향(0~Tmax)이므로 음수는 0으로
    u = max(u, 0);
    u = min(u, Tmax);

    F_ach = B*u;
end


function pwm = thrust_to_pwm(u, Tmax, pwmMax, pwmMin)
    % u: Nx1 thrust command [N]
    % pwmMax: 예) 65535 또는 255
    % pwmMin: (선택) 밸브/드라이버가 실제로 열리는 최소 duty가 있으면 반영

    duty = u(:) / Tmax;          % 0~1
    duty = max(0, min(1, duty));

    if nargin >= 4 && pwmMin > 0
        % duty>0인 경우에만 최소 구동 듀티 적용(데드존)
        duty(duty>0) = max(duty(duty>0), pwmMin/pwmMax);
    end

    pwm = round(duty * pwmMax);
end
